simulink model "test"  (R2024b)
settings: Solver=VariableStepAuto  StartTime=0.0  StopTime=10.0  RelTol=1e-3
settings Model: Creator=wolfl  LastModifiedBy=wolfl

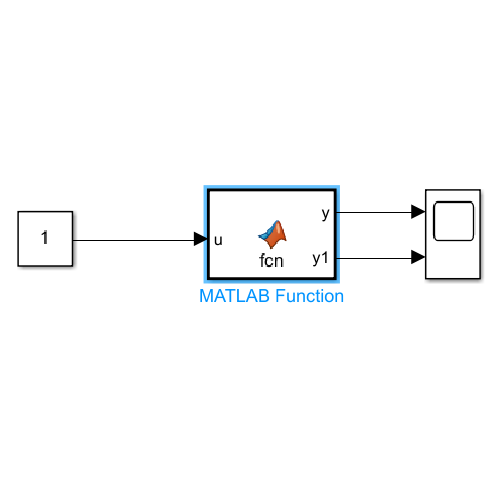
[thumbnail: Simulink's stored preview of the top-level diagram]
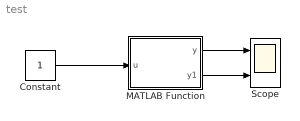
== system test ==
  Constant : Constant
  MATLAB Function : MATLAB Function  TreatAsAtomicUnit=on
  Scope : Scope  NumInputPorts=2
  wires:
  Constant/1 -> MATLAB Function/1(u)
  MATLAB Function/1(y) -> Scope/1
  MATLAB Function/2(y1) -> Scope/2

== matlab function test/MATLAB Function ==
  data: u input; y output; Q parameter; y1 output
function [y, y1] = fcn(u, Q)

x = Q(1,1)*10^5;

y = u + x;
y1 = x;
